simulink model "FLC_PI"  (R2022a)
settings: Solver=VariableStepAuto  StartTime=0.0  StopTime=20  RelTol=1e-3
model workspace (MAT data in the model file):
  fuzzy : mamfis (value not decoded)
libraries: fuzblock x1
settings Model: Creator=Ελένη  LastModifiedBy=Ελένη

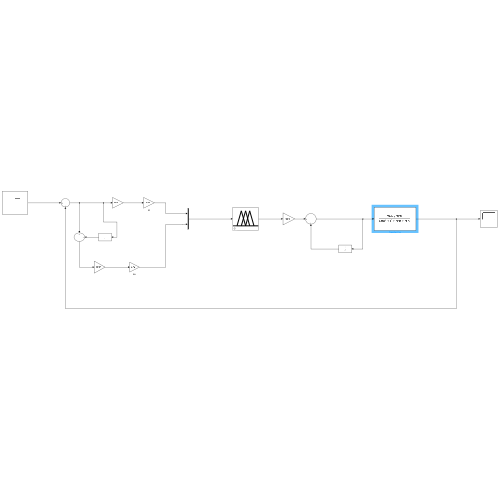
[thumbnail: Simulink's stored preview of the top-level diagram]
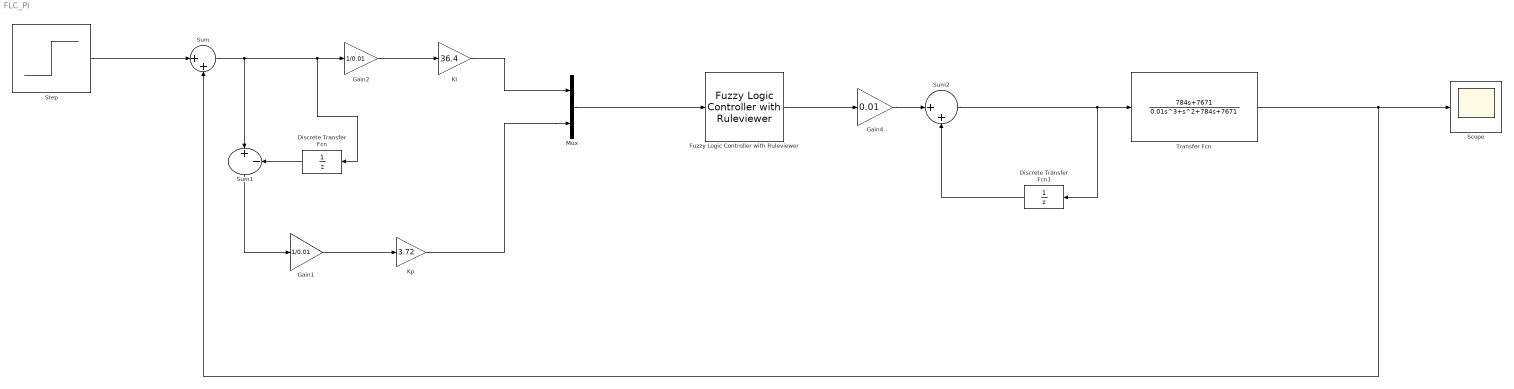
== system FLC_PI ==
  Discrete Transfer Fcn : DiscreteTransferFcn  Denominator=[1 0]
  Discrete Transfer Fcn1 : DiscreteTransferFcn  Denominator=[1 0]
  Fuzzy Logic Controller with Ruleviewer : fuzblock/Fuzzy Logic  Controller  with Ruleviewer  fismatrix=fuzzy  Ts=2
  Gain1 : Gain  Gain=1/0.01
  Gain2 : Gain  Gain=1/0.01
  Gain4 : Gain  Gain=0.01
  KI : Gain  Gain=36.4
  Kp : Gain  Gain=3.72
  Mux : Mux  Inputs=2
  Scope : Scope
  Step : Step  Time=0.01  SampleTime=0
  Sum : Sum  Inputs=|++
  Sum1 : Sum  Inputs=|+-
  Sum2 : Sum  Inputs=|++
  Transfer Fcn : TransferFcn  Numerator=[784 7671]  Denominator=[0.01 1 784 7671]
  wires:
  Step/1 -> Sum/1
  Gain2/1 -> KI/1
  KI/1 -> Mux/1
  Sum/1 -> Sum1/1, Discrete Transfer Fcn/1, Gain2/1
  Discrete Transfer Fcn/1 -> Sum1/2
  Sum1/1 -> Gain1/1
  Gain1/1 -> Kp/1
  Kp/1 -> Mux/2
  Gain4/1 -> Sum2/1
  Discrete Transfer Fcn1/1 -> Sum2/2
  Sum2/1 -> Discrete Transfer Fcn1/1, Transfer Fcn/1
  Transfer Fcn/1 -> Scope/1, Sum/2
  Mux/1 -> Fuzzy Logic Controller with Ruleviewer/1
  Fuzzy Logic Controller with Ruleviewer/1 -> Gain4/1
